simulink library "toPDB"  (R2016b)
settings: Solver=VariableStepAuto  StartTime=0.0  StopTime=10.0  RelTol=1e-3
settings Model: Creator=Nathan  LastModifiedBy=march

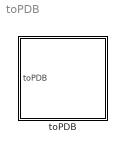
== system toPDB ==
  toPDB : Subsystem

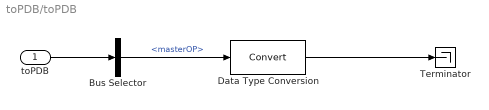
== system toPDB/toPDB ==
  toPDB : Inport  OutDataTypeStr=Bus: toPDB  BusOutputAsStruct=on
  Bus Selector : BusSelector  OutputSignals=masterOP
  Data Type Conversion : DataTypeConversion
  Terminator : Terminator
  wires:
  Data Type Conversion/1 -> Terminator/1
  Bus Selector/1 -> Data Type Conversion/1  "<masterOP>"
  toPDB/1 -> Bus Selector/1
